simulink model "process_plant_model"  (R2020a)
settings: Solver=VariableStepAuto  StartTime=0.0  StopTime=2500  RelTol=1e-3
values from neighbouring files (symbols this model uses):
  B = [b11 b12 b13 b14 b15 b16 ... (first row only)    [constants.m]    (also in constants_dp_model.m; constants_model_coriolis.m; constants_process_model.m)
  B_psinv_law = B_law'/(B_law*B_law')    [constants_process_model.m]
  D = diag([d_11 d_22 d_33 d_44 d_55 d_66])    [constants.m]    (also in constants_dp_model.m = diag([d_11 d_22 d_33 d_44]); constants_model_coriolis.m = diag([d_11 d_22 d_33 d_44]); constants_process_model.m)
  eta0 = [x0; y0; z0; phi0; theta0; psi0]    [constants.m]    (also in constants_dp_model.m = [x0; y0; z0; psi0]; constants_model_coriolis.m = [x0; y0; z0; psi0]; constants_process_model.m)
  M_A = diag([m_A11 m_A22 m_A33 m_A44 m_A55 m_A66])    [constants.m]    (also in constants_dp_model.m = diag([m_A11 m_A22 m_A33 m_A44]); constants_model_coriolis.m = diag([m_A11 m_A22 m_A33 m_A44]); constants_process_model.m)
  M_inv = inv(M)    [constants.m]    (also in constants_process_model.m)
  ny0 = [u0; v0; w0; p0; q0; r0]    [constants.m]    (also in constants_dp_model.m = [u0; v0; w0; r0]; constants_model_coriolis.m = [u0; v0; w0; r0]; constants_process_model.m)
  V_x = 1    [constants.m]    (also in constants_process_model.m; run_simulation_FL_controller.m = 0.25; run_simulation_PID_controller.m = 0.25; run_simulation_dp_model.m = 0.25)
  V_y = 0    [constants.m]    (also in constants_process_model.m; run_simulation_FL_controller.m = -0.6; run_simulation_PID_controller.m = -0.6; run_simulation_dp_model.m = -0.6)
settings Model: Creator=kenng  LastModifiedBy=kenng

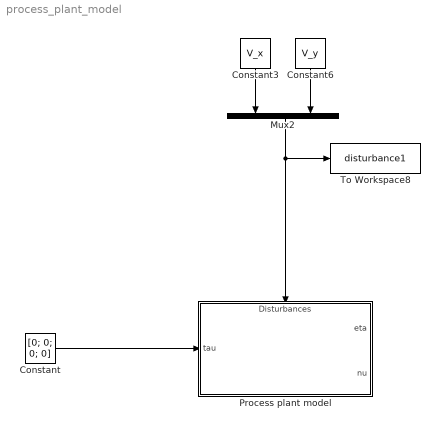
== system process_plant_model ==
  Constant : Constant  Value=[0; 0; 0; 0]
  Constant3 : Constant  Value=V_x
  Constant6 : Constant  Value=V_y
  Mux2 : Mux  Inputs=2
  Process plant model : Subsystem
      settings: PortSchema="{\"entries\":[{\"content\":{\"sides\":[{\"content\":{\"connectorIds\":[\"In1\"]},\"type\":\"ConnectorPlacement.EquallySpacedRectSide\",\"uuid\":\"730cb069-5b49-459f-9304-e4a866821db5\"},{\"content\":{\"connectorIds\":[\"Out1\",\"Out2\"],\"side\":\"RIGHT\"},\"type\":\"ConnectorPlacement.EquallySpacedRectSide\",\"uuid\":\"42a5cffb-0e0b-4bb5-858a-ba08346c14eb\"},{\"content\":{\"connectorIds\":[\"In2\"],\"side\":\"TOP\"},\"type\":\"ConnectorPlacement.EquallySpacedRectSide\",\"uuid\":\"204f6fa7-c975-425d-92ff-491a236dd291\"}]},\"type\":\"ConnectorPlacement.EquallySpacedConnector\",\"uuid\":\"abcefe49-80f8-40a8-906d-9a8c96e17f4b\"}],\"packageUris\":[\"http://schema.mathworks.com/mf0/Connector/19700101\"],\"version\":\"1.0\"}"
  To Workspace8 : ToWorkspace  VariableName=disturbance1  SaveFormat=Structure With Time  SampleTime=-1
  wires:
  Constant3/1 -> Mux2/1
  Constant6/1 -> Mux2/2
  Mux2/1 -> Process plant model/2(Disturbances), To Workspace8/1
  Constant/1 -> Process plant model/1(tau)

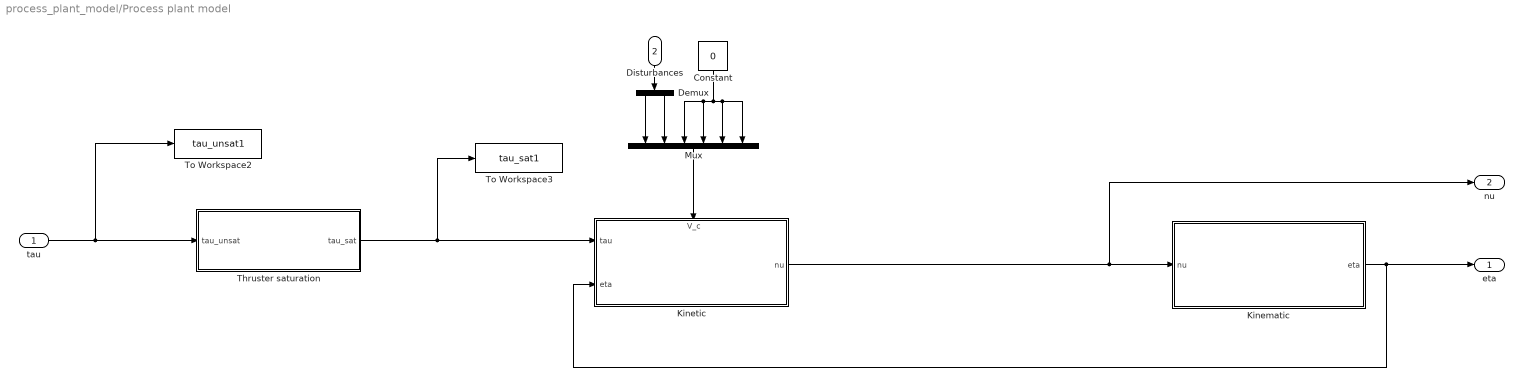
== system process_plant_model/Process plant model ==
  tau : Inport
  Disturbances : Inport  Port=2
  Constant : Constant  Value=0
  Demux : Demux  Outputs=2
  Kinematic : Subsystem
  Kinetic : Subsystem
      settings: PortSchema="{\"entries\":[{\"content\":{\"sides\":[{\"content\":{\"connectorIds\":[\"In1\",\"In2\"]},\"type\":\"ConnectorPlacement.EquallySpacedRectSide\",\"uuid\":\"0179b693-99c9-4769-8568-748fff456238\"},{\"content\":{\"connectorIds\":[\"Out1\"],\"side\":\"RIGHT\"},\"type\":\"ConnectorPlacement.EquallySpacedRectSide\",\"uuid\":\"7327462f-f467-4f02-8532-f5a0a2ed6492\"},{\"content\":{\"connectorIds\":[\"In3\"],\"side\":\"TOP\"},\"type\":\"ConnectorPlacement.EquallySpacedRectSide\",\"uuid\":\"2b2eda63-e901-4425-a94a-dc361cab137d\"}]},\"type\":\"ConnectorPlacement.EquallySpacedConnector\",\"uuid\":\"fa1c0f5e-2991-4de2-ab09-c8d1308c5531\"}],\"packageUris\":[\"http://schema.mathworks.com/mf0/Connector/19700101\"],\"version\":\"1.0\"}"
  Mux : Mux  Inputs=6
  Thruster saturation : Subsystem
  To Workspace2 : ToWorkspace  VariableName=tau_unsat1  SaveFormat=Structure With Time  SampleTime=-1
  To Workspace3 : ToWorkspace  VariableName=tau_sat1  SaveFormat=Structure With Time  SampleTime=-1
  eta : Outport
  nu : Outport  Port=2
  wires:
  Kinetic/1(nu) -> nu/1, Kinematic/1(nu)
  Kinematic/1(eta) -> Kinetic/2(eta), eta/1
  Disturbances/1 -> Demux/1
  Demux/1 -> Mux/1
  Demux/2 -> Mux/2
  Constant/1 -> Mux/3, Mux/4, Mux/6, Mux/5
  Mux/1 -> Kinetic/3(V_c)
  tau/1 -> To Workspace2/1, Thruster saturation/1(tau_unsat)
  Thruster saturation/1(tau_sat) -> To Workspace3/1, Kinetic/1(tau)

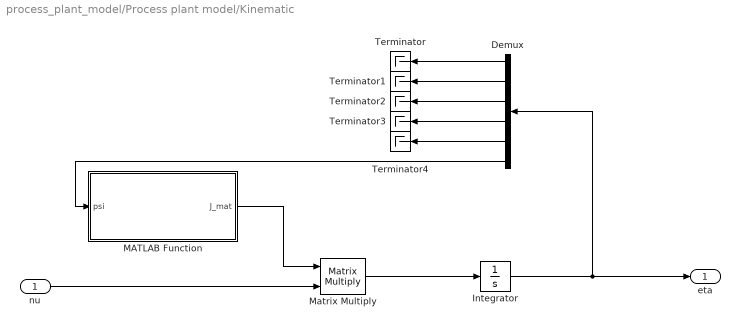
== system process_plant_model/Process plant model/Kinematic ==
  nu : Inport
  Demux : Demux  Outputs=6
  Integrator : Integrator  InitialCondition=eta0
  MATLAB Function : MATLAB Function  TreatAsAtomicUnit=on
  Matrix Multiply : Product  Multiplication=Matrix(*)
  Terminator{,1..4} (5 alike) : Terminator
  eta : Outport
  wires:
  Integrator/1 -> Demux/1, eta/1
  Demux/6 -> MATLAB Function/1(psi)
  Demux/1 -> Terminator/1
  Demux/2 -> Terminator1/1
  Demux/3 -> Terminator2/1
  Demux/4 -> Terminator3/1
  Demux/5 -> Terminator4/1
  MATLAB Function/1(J_mat) -> Matrix Multiply/1
  nu/1 -> Matrix Multiply/2
  Matrix Multiply/1 -> Integrator/1

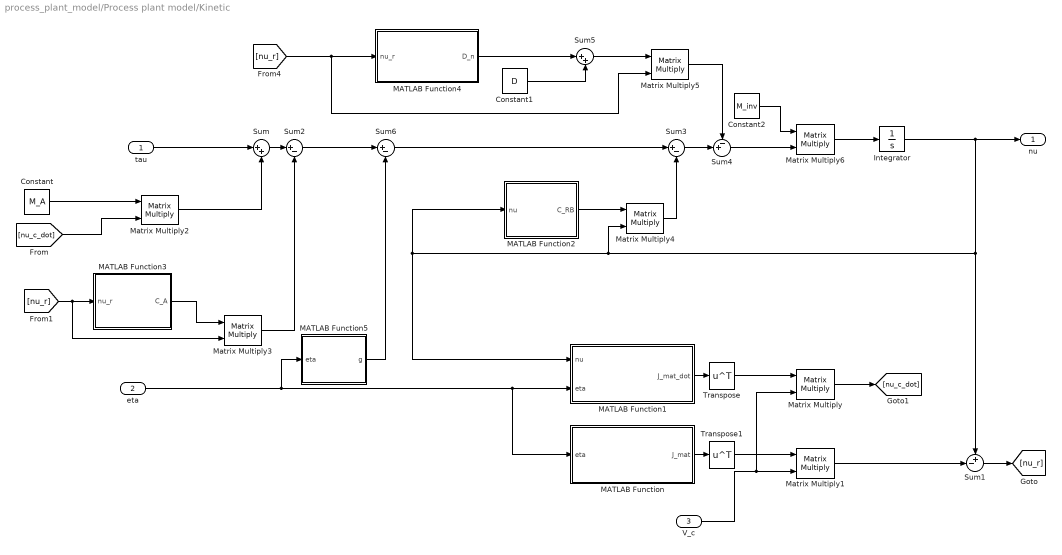
== system process_plant_model/Process plant model/Kinetic ==
  tau : Inport
  eta : Inport  Port=2
  V_c : Inport  Port=3
  Constant : Constant  Value=M_A
  Constant1 : Constant  Value=D
  Constant2 : Constant  Value=M_inv
  Integrator : Integrator  InitialCondition=ny0
  MATLAB Function : MATLAB Function  TreatAsAtomicUnit=on
  MATLAB Function1 : MATLAB Function  TreatAsAtomicUnit=on
  MATLAB Function2 : MATLAB Function  TreatAsAtomicUnit=on
  MATLAB Function3 : MATLAB Function  TreatAsAtomicUnit=on
  MATLAB Function4 : MATLAB Function  TreatAsAtomicUnit=on
  MATLAB Function5 : MATLAB Function  TreatAsAtomicUnit=on
  Matrix Multiply{,1..6} (7 alike) : Product  Multiplication=Matrix(*)
  Sum : Sum  Inputs=|++
  Sum1 : Sum  Inputs=+-|
  Sum2 : Sum  Inputs=|+-
  Sum3 : Sum  Inputs=|+-
  Sum4 : Sum  Inputs=-+|
  Sum5 : Sum  Inputs=|++
  Sum6 : Sum  Inputs=|+-
  Transpose : Math  Operator=transpose  SaturateOnIntegerOverflow=on
  Transpose1 : Math  Operator=transpose  SaturateOnIntegerOverflow=on
  nu : Outport
  wires:
  Integrator/1 -> MATLAB Function2/1(nu), MATLAB Function1/1(nu), Matrix Multiply4/2, Sum1/1, nu/1
  eta/1 -> MATLAB Function5/1(eta), MATLAB Function/1(eta), MATLAB Function1/2(eta)
  MATLAB Function/1(J_mat) -> Transpose1/1
  MATLAB Function1/1(J_mat_dot) -> Transpose/1
  V_c/1 -> Matrix Multiply1/2, Matrix Multiply/2
  Transpose/1 -> Matrix Multiply/1
  Transpose1/1 -> Matrix Multiply1/1
  Matrix Multiply/1 -> [nu_c_dot]
  Matrix Multiply1/1 -> Sum1/2
  Sum1/1 -> [nu_r]
  tau/1 -> Sum/1
  Constant/1 -> Matrix Multiply2/1
  [nu_c_dot] -> Matrix Multiply2/2
  Matrix Multiply2/1 -> Sum/2
  [nu_r] -> Matrix Multiply3/2, MATLAB Function3/1(nu_r)
  MATLAB Function3/1(C_A) -> Matrix Multiply3/1
  Sum/1 -> Sum2/1
  Matrix Multiply3/1 -> Sum2/2
  MATLAB Function2/1(C_RB) -> Matrix Multiply4/1
  Matrix Multiply4/1 -> Sum3/2
  [nu_r] -> MATLAB Function4/1(nu_r), Matrix Multiply5/2
  MATLAB Function4/1(D_n) -> Sum5/1
  Constant1/1 -> Sum5/2
  Sum5/1 -> Matrix Multiply5/1
  Sum3/1 -> Sum4/2
  Matrix Multiply5/1 -> Sum4/1
  Sum2/1 -> Sum6/1
  Sum6/1 -> Sum3/1
  MATLAB Function5/1(g) -> Sum6/2
  Sum4/1 -> Matrix Multiply6/2
  Constant2/1 -> Matrix Multiply6/1
  Matrix Multiply6/1 -> Integrator/1

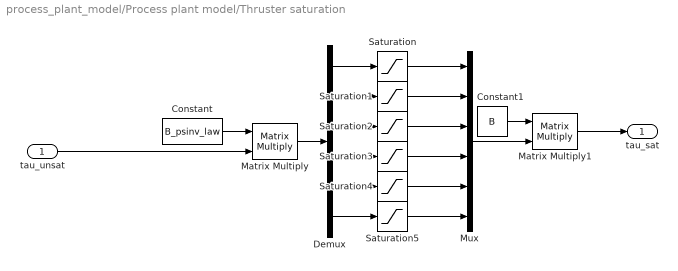
== system process_plant_model/Process plant model/Thruster saturation ==
  tau_unsat : Inport
  Constant : Constant  Value=B_psinv_law
  Constant1 : Constant  Value=B
  Demux : Demux  Outputs=6
  Matrix Multiply : Product  Multiplication=Matrix(*)
  Matrix Multiply1 : Product  Multiplication=Matrix(*)
  Mux : Mux  Inputs=6
  Saturation{,1..5} (6 alike) : Saturate  UpperLimit=120  LowerLimit=-120
  tau_sat : Outport
  wires:
  tau_unsat/1 -> Matrix Multiply/2
  Constant/1 -> Matrix Multiply/1
  Matrix Multiply/1 -> Demux/1
  Demux/2 -> Saturation1/1
  Demux/1 -> Saturation/1
  Demux/3 -> Saturation2/1
  Demux/4 -> Saturation3/1
  Demux/5 -> Saturation4/1
  Demux/6 -> Saturation5/1
  Saturation/1 -> Mux/1
  Saturation1/1 -> Mux/2
  Saturation2/1 -> Mux/3
  Saturation3/1 -> Mux/4
  Saturation4/1 -> Mux/5
  Saturation5/1 -> Mux/6
  Mux/1 -> Matrix Multiply1/2
  Constant1/1 -> Matrix Multiply1/1
  Matrix Multiply1/1 -> tau_sat/1

== matlab function process_plant_model/Process plant model/Kinetic/MATLAB Function ==
  data: eta input size=[6 1]; J_mat output size=[6 6]
function J_mat = transformation_matrix(eta)
%#codegen
    psi   = eta(6);
    J_mat = [cos(psi) -sin(psi) 0 0 0 0;
            sin(psi) cos(psi) 0 0 0 0;
            0 0 1 0 0 0;
            0 0 0 1 0 0;
            0 0 0 0 1 0;
            0 0 0 0 0 1];

== matlab function process_plant_model/Process plant model/Kinetic/MATLAB Function1 ==
  data: nu input size=[6 1]; eta input size=[6 1]; J_mat_dot output size=[6 6]
function J_mat_dot = transformation_matrix_dot(nu, eta)
%#codegen
    psi         = eta(6);
    r           = nu(6);
    J_mat_dot   = [-r*sin(psi) -r*cos(psi) 0 0 0 0;
                    r*cos(psi) -r*sin(psi) 0 0 0 0;
                    0 0 0 0 0 0;
                    0 0 0 0 0 0;
                    0 0 0 0 0 0;
                    0 0 0 0 0 0];

== matlab function process_plant_model/Process plant model/Kinetic/MATLAB Function2 ==
  data: nu input size=[6 1]; C_RB output size=[6 6]
function C_RB = coriolis_rb(nu)
%#codegen
    u       = nu(1);
    v       = nu(2);
    w       = nu(3);
    p       = nu(4);
    q       = nu(5);
    r       = nu(6);

    C_RB    = [0 0 0 0 450*w -162*v;
                0 0 0 -450*w 0 144*u;
                0 0 0 162*v -144*u-r 0;
                0 450*w -162*v 0 18.2*r -66.5*q;
                -450*w 0 144*u -18.2*r 0 21*p;
                162*v -144*u 0 66.5*q -21*p 0];

== matlab function process_plant_model/Process plant model/Kinetic/MATLAB Function3 ==
  data: nu_r input size=[6 1]; C_A output size=[6 6]
function C_A = coriolis_A(nu_r)
%#codegen
    
    u_r     = nu_r(1);
    v_r     = nu_r(2);
    w_r     = nu_r(3);
    p_r     = nu_r(4);
    q_r     = nu_r(5);
    r_r     = nu_r(6);

    C_A     = [0 0 0 0 450*w_r -162*v_r;
                0 0 0 -450*w_r 0 144*u_r;
                0 0 0 162*v_r -144*u_r 0;
                0 450*w_r -162*v_r 0 18.2*r_r -66.5*q_r;
                -450*w_r 0 144*u_r -18.2*r_r 0 21*p_r;
                162*v_r -144*u_r 0 66.5*q_r -21*p_r 0];

== matlab function process_plant_model/Process plant model/Kinetic/MATLAB Function4 ==
  data: nu_r input size=[6 1]; D_n output size=[6 6]
function D_n = damping_n(nu_r)
%#codegen
    u_r     = nu_r(1);
    v_r     = nu_r(2);
    w_r     = nu_r(3);
    p_r     = nu_r(4);
    q_r     = nu_r(5);
    r_r     = nu_r(6);
    
    D_n     = [350*abs(u_r) 0 0 0 0 0;
                0 350*abs(v_r) 0 0 0 0;
                0 0 400*abs(w_r) 0 0 0;
                0 0 0 100*abs(p_r) 0 0;
                0 0 0 0 100*abs(q_r) 0;
                0 0 0 0 0 75*abs(r_r)];

== matlab function process_plant_model/Process plant model/Kinetic/MATLAB Function5 ==
  data: eta input size=[6 1]; g output size=[6 1]
function g = restoring_forces(eta)
%#codegen
    phi     = eta(4);
    theta   = eta(5);
    
    g       = [-0.91*sin(theta);
                0.91*cos(theta)*sin(phi);
                0.91*cos(theta)*cos(phi);
                0.18*cos(theta)*sin(phi);
                0.18*sin(theta);
                0];

== matlab function process_plant_model/Process plant model/Kinematic/MATLAB Function ==
  data: psi input size=[1]; J_mat output size=[6 6]
function J_mat = transformation_matrix(psi)
%#codegen
    J_mat = [cos(psi) -sin(psi) 0 0 0 0;
            sin(psi) cos(psi) 0 0 0 0;
            0 0 1 0 0 0;
            0 0 0 1 0 0;
            0 0 0 0 1 0;
            0 0 0 0 0 1];
